simulink model "Noa_Nofusion"  (R2020b)
settings: Solver=FixedStepDiscrete  StartTime=0.0  StopTime=Inf  FixedStep=0.01  RelTol=1e-3
PostLoadFcn:
  | if any(exist('dsrtsu_mdlpostloadfcn', 'file') ~= 0), dsrtsu_mdlpostloadfcn('Execute', bdroot); end
InitFcn:
  | , if any(exist('rtifpga_mdlclblib', 'file') ~= 0), rtifpga_mdlclblib('Init', bdroot); end,
  | , if any(exist('dsmpb_private', 'file') ~= 0), dsmpb_private('dsmpb_mdlclblib', 'Init', bdroot); end,
undefined symbols (not defined in the file or in its folder): ACC_TimeGap_DecSetSwt, ACC_TimeGap_IncSetSwt, AccelPedalPosn, AccelPedalPosnVldty, AccelPedlPosnDiagc, AccPedalOverride, ACU_ShiftInProgress, ADAS_Posn_CurLane, AESSwtReq, ALC_SwtReq, BrkPedalSts, CC_ACC_CANCEL_OFFSwt, CC_ACC_CRUISE_OFFSwt, CC_ACC_DecSetSpd_SetSwt, CC_ACC_IncSetSpd_ResuSwt, CC_ACCSwtErr, CharSpd_ms, CSA_NODE, CURRENT_GEAR, CurrentGearValid, DiscIntNeverNeededParam, DrvDoorSts, DrvSBR, DrvTrqReqOvld, ECMACCInterface, ECMRespACC, ELKSwtReq, EngLimpHomeSts, EngSpd, EngState, EngState_PHEV, EngTrqMaxActSpd, EngTrqMinAct, EPS_DrvInpTrqVal_HighReslolution, EPS_FailSts, EPS_LKATorqOvrlDlvd, EPS_LKATorqOvrlDlvdVld, EPS_LKATrqOvlDlvdSts, EPS_SteerMod, EPS_TrqSnsrSts, EQ4_APPINFO, EQ4_LA_ELEM, EQ4_LA_HDR, EQ4_LAP_ELEM, EQ4_LAP_HDR, EQ4_LH_ELEM, EQ4_LH_HDR, EQ4_LRE_ELEM, EQ4_LRE_HDR, ESS_PedSwtReq, ESS_VehSwtReq, FFogLmpSts_F_Pbox, FLWheelDriveDirection, FLWheelSpd, FrntWiprSwtSts, FrntWshrSwtSts, FRWheelDriveDirection, FRWheelSpd, HazardLmpSwtSts, HCU_AccelPedalPosn_Diag ... (+151)
libraries: simulink x144, dsmpblib x33, canfdmsglib x10
(part 14 of 20)

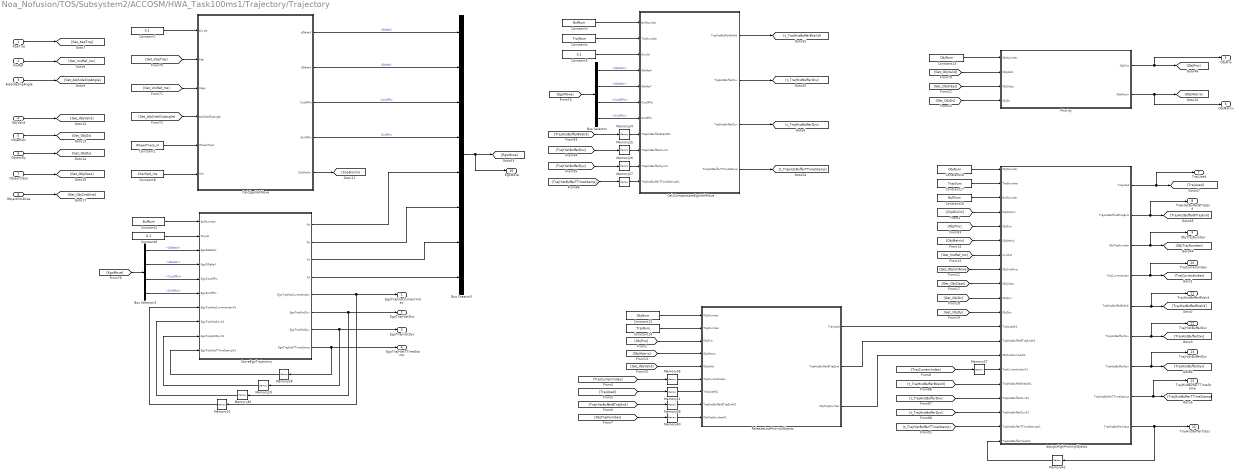
== system Noa_Nofusion/TOS/Subsystem2/ACCOSM/HWA_Task100ms1/Trajectory/Trajectory ==
  KapTraj : Inport
  VxvRef : Inport  Port=2
  AlpSideSlipAngle : Inport  Port=3
  ObjValid : Inport  Port=4
  ObjectDx : Inport  Port=5
  ObjectDy : Inport  Port=6
  ObjectClass : Inport  Port=7
  ObjectCntAlive : Inport  Port=8
  AssignHighPriorityObjects : MATLAB Function  TreatAsAtomicUnit=on
  Bus Creator3 : BusCreator  Inputs=8
  Bus Selector : BusSelector  OutputSignals=dDeltaX,dDeltaY,CosOfPsi,SinOfPsi
  Bus Selector3 : BusSelector  OutputSignals=dDeltaX,dDeltaY,CosOfPsi,SinOfPsi
  CalcCompensateEgoVehMove : MATLAB Function  TreatAsAtomicUnit=on
  CalcEgoVehMove : MATLAB Function  TreatAsAtomicUnit=on
  Constant1 : Constant  Value=WheelTrack_m  OutDataTypeStr=single
  Constant13 : Constant  Value=ObjNum  OutDataTypeStr=uint8
  Constant14 : Constant  Value=TrajNum  OutDataTypeStr=uint8
  Constant15 : Constant  Value=ObjNum  OutDataTypeStr=uint8
  Constant16 : Constant  Value=BufNum  OutDataTypeStr=uint8
  Constant17 : Constant  Value=TrajNum  OutDataTypeStr=uint8
  Constant18 : Constant  Value=ObjNum  OutDataTypeStr=uint8
  Constant2 : Constant  Value=BufNum  OutDataTypeStr=uint8
  Constant3 : Constant  Value=BufNum  OutDataTypeStr=uint8
  Constant4 : Constant  Value=TrajNum  OutDataTypeStr=uint8
  Constant5 : Constant  Value=0.1  OutDataTypeStr=single
  Constant6 : Constant  Value=0.1  OutDataTypeStr=single
  Constant7 : Constant  Value=0.1  OutDataTypeStr=single
  Constant8 : Constant  Value=CharSpd_ms  OutDataTypeStr=single
  Memory{24..26,42} (4 alike) : Memory  InitialCondition=zeros(TrajNum,BufNum)  InheritSampleTime=on
  Memory27 : Memory  InitialCondition=32*ones(TrajNum,BufNum)  InheritSampleTime=on
  Memory28 : Memory  InitialCondition=32*ones(BufNum,1)  InheritSampleTime=on
  Memory29 : Memory  InitialCondition=zeros(BufNum,1)  InheritSampleTime=on
  Memory30 : Memory  InitialCondition=zeros(BufNum,1)  InheritSampleTime=on
  Memory31 : Memory  InitialCondition=1  InheritSampleTime=on
  Memory36 : Memory  InitialCondition=ones(TrajNum,1)  InheritSampleTime=on
  Memory37 : Memory  InitialCondition=ones(TrajNum,1)  InheritSampleTime=on
  Memory38 : Memory  InitialCondition=ones(TrajNum,BufNum)  InheritSampleTime=on
  Memory40 : Memory  InitialCondition=255*ones(ObjNum,1)  InheritSampleTime=on
  Memory41 : Memory  InitialCondition=zeros(TrajNum,1)  InheritSampleTime=on
  Priority : MATLAB Function  TreatAsAtomicUnit=on
  ReleaseLowPriorityObjects : MATLAB Function  TreatAsAtomicUnit=on
  StoreEgoTrajectory : MATLAB Function  TreatAsAtomicUnit=on
  EgoTrajHistCurrentIndex : Outport
  EgoTrajHistDxv : Outport  Port=2
  EgoTrajHistDyv : Outport  Port=3
  EgoTrajHistTTimeStamp : Outport  Port=4
  ObjPrio : Outport  Port=5
  ObjMatrix : Outport  Port=6
  TrajUsed : Outport  Port=7
  TrajHistBufferBTrajEnd : Outport  Port=8
  ObjTrajNumber : Outport  Port=9
  TrajCurrentIndex : Outport  Port=10
  TrajHistBufferBValid : Outport  Port=11
  TrajHistBufferDxv : Outport  Port=12
  TrajHistBufferDyv : Outport  Port=13
  TrajHistBufferTTimeStamp : Outport  Port=14
  TrajHistBufferClass : Outport  Port=15
  EgoMove : Outport  Port=16
  wires:
  StoreEgoTrajectory/1(Pa) -> Bus Creator3/5
  StoreEgoTrajectory/2(Pb) -> Bus Creator3/6
  StoreEgoTrajectory/3(Pc) -> Bus Creator3/7
  StoreEgoTrajectory/4(Pd) -> Bus Creator3/8
  Bus Creator3/1 -> [EgoMove], EgoMove/1
  [SlipDislim] -> AssignHighPriorityObjects/4(SlipDisLim)
  CalcEgoVehMove/5(SlipDislim) -> [SlipDislim]
  Constant8/1 -> CalcEgoVehMove/6(Vch)
  Constant1/1 -> CalcEgoVehMove/5(WheelTrack)
  CalcCompensateEgoVehMove/3(TrajHistBufferDyv) -> [t_TrajHistBufferDyv]
  Priority/2(ObjMatrix) -> ObjMatrix/1, [ObjMatrix]
  Priority/1(ObjPrio) -> [ObjPrio], ObjPrio/1
  CalcEgoVehMove/4(SinOfPsi) -> Bus Creator3/4  "SinOfPsi"
  CalcEgoVehMove/3(CosOfPsi) -> Bus Creator3/3  "CosOfPsi"
  CalcEgoVehMove/2(dDeltaY) -> Bus Creator3/2  "dDeltaY"
  CalcEgoVehMove/1(dDeltaX) -> Bus Creator3/1  "dDeltaX"
  ObjectCntAlive/1 -> [Get_ObjCntAlive]
  ObjectClass/1 -> [Get_ObjClass]
  ObjectDx/1 -> [Get_ObjDx]
  ObjectDy/1 -> [Get_ObjDy]
  ObjValid/1 -> [Get_ObjValid]
  AssignHighPriorityObjects/8(TrajHistBufferTTimeStamp) -> [TrajHistBufferTTimeStamp], TrajHistBufferTTimeStamp/1
  Bus Selector3/1 -> StoreEgoTrajectory/3(EgoDDeltaX)  "<dDeltaX>"
  Bus Selector3/4 -> StoreEgoTrajectory/6(EgoSinOfPsi)  "<SinOfPsi>"
  Bus Selector3/2 -> StoreEgoTrajectory/4(EgoDDeltaY)  "<dDeltaY>"
  Bus Selector3/3 -> StoreEgoTrajectory/5(EgoCosOfPsi)  "<CosOfPsi>"
  StoreEgoTrajectory/8(EgoTrajHistTTimeStamp) -> Memory28/1, EgoTrajHistTTimeStamp/1
  Memory31/1 -> StoreEgoTrajectory/7(EgoTrajHistCurrentIndexK1)
  StoreEgoTrajectory/5(EgoTrajHistCurrentIndex) -> Memory31/1, EgoTrajHistCurrentIndex/1
  Memory30/1 -> StoreEgoTrajectory/8(EgoTrajHistDxvK1)
  StoreEgoTrajectory/6(EgoTrajHistDxv) -> Memory30/1, EgoTrajHistDxv/1
  Memory29/1 -> StoreEgoTrajectory/9(EgoTrajHistDyvK1)
  Memory28/1 -> StoreEgoTrajectory/10(EgoTrajHistTTimeStampK1)
  StoreEgoTrajectory/7(EgoTrajHistDyv) -> Memory29/1, EgoTrajHistDyv/1
  Constant6/1 -> StoreEgoTrajectory/2(tCycle)
  Constant2/1 -> StoreEgoTrajectory/1(BufNumber)
  [ObjMatrix] -> AssignHighPriorityObjects/6(ObjMatrix)
  [ObjMatrix] -> ReleaseLowPriorityObjects/4(ObjMatrix)
  Constant16/1 -> AssignHighPriorityObjects/3(BufNumber)
  Constant17/1 -> AssignHighPriorityObjects/2(TrajNumber)
  Constant18/1 -> AssignHighPriorityObjects/1(ObjNumber)
  Constant14/1 -> ReleaseLowPriorityObjects/2(TrajNumber)
  Constant15/1 -> ReleaseLowPriorityObjects/1(ObjNumber)
  Constant13/1 -> Priority/1(ObjNumber)
  Constant4/1 -> CalcCompensateEgoVehMove/2(TrajNumber)
  Constant3/1 -> CalcCompensateEgoVehMove/1(BufNumber)
  AlpSideSlipAngle/1 -> [Get_AlpSideSlipAngle]
  VxvRef/1 -> [Get_VxvRef_ms]
  KapTraj/1 -> [Get_KapTraj]
  [Get_ObjCntAlive] -> AssignHighPriorityObjects/8(ObjCntAlive)
  [TrajHistBufferBValid] -> Memory24/1
  [TrajHistBufferDyv] -> Memory26/1
  [TrajHistBufferDxv] -> Memory25/1
  [TrajHistBufferTTimeStamp] -> Memory27/1
  [Get_ObjDy] -> AssignHighPriorityObjects/11(ObjDyv)
  AssignHighPriorityObjects/4(TrajCurrentIndex) -> [TrajCurrentIndex], TrajCurrentIndex/1
  [Get_ObjDx] -> AssignHighPriorityObjects/10(ObjDxv)
  [Get_ObjClass] -> AssignHighPriorityObjects/9(ObjClass)
  [Get_VxvRef_ms] -> AssignHighPriorityObjects/7(VxvRef)
  [TrajCurrentIndex] -> Memory37/1
  [TrajCurrentIndex] -> Memory36/1
  AssignHighPriorityObjects/6(TrajHistBufferDxv) -> [TrajHistBufferDxv], TrajHistBufferDxv/1
  AssignHighPriorityObjects/7(TrajHistBufferDyv) -> [TrajHistBufferDyv], TrajHistBufferDyv/1
  AssignHighPriorityObjects/5(TrajHistBufferBValid) -> [TrajHistBufferBValid], TrajHistBufferBValid/1
  [Get_ObjValid] -> ReleaseLowPriorityObjects/5(ObjValid)
  [ObjPrio] -> ReleaseLowPriorityObjects/3(ObjPrio)
  [TrajHistBufferBTrajEnd] -> Memory38/1
  [ObjTrajNumber] -> Memory40/1
  [TrajUsed] -> Memory41/1
  Memory42/1 -> AssignHighPriorityObjects/20(TrajHistBufferClassK1)
  Memory41/1 -> ReleaseLowPriorityObjects/7(TrajUsedK1)
  Memory40/1 -> ReleaseLowPriorityObjects/9(ObjTrajNumberK1)
  Memory38/1 -> ReleaseLowPriorityObjects/8(TrajHistBufferBTrajEndK1)
  Memory37/1 -> AssignHighPriorityObjects/15(TrajCurrentIndexK1)
  Memory36/1 -> ReleaseLowPriorityObjects/6(TrajCurrentIndex)
  [t_TrajHistBufferTTimeStamp] -> AssignHighPriorityObjects/19(TrajHistBufferTTimeStampK1)
  CalcCompensateEgoVehMove/4(TrajHistBufferTTimeStamp) -> [t_TrajHistBufferTTimeStamp]
  [t_TrajHistBufferDyv] -> AssignHighPriorityObjects/18(TrajHistBufferDyvK1)
  [t_TrajHistBufferDxv] -> AssignHighPriorityObjects/17(TrajHistBufferDxvK1)
  CalcCompensateEgoVehMove/2(TrajHistBufferDxv) -> [t_TrajHistBufferDxv]
  [t_TrajHistBufferBValid] -> AssignHighPriorityObjects/16(TrajHistBufferBValidK1)
  CalcCompensateEgoVehMove/1(TrajHistBufferBValid) -> [t_TrajHistBufferBValid]
  [ObjPrio] -> AssignHighPriorityObjects/5(ObjPrio)
  AssignHighPriorityObjects/9(TrajHistBufferClass) -> TrajHistBufferClass/1, Memory42/1
  AssignHighPriorityObjects/2(TrajHistBufferBTrajEnd) -> [TrajHistBufferBTrajEnd], TrajHistBufferBTrajEnd/1
  AssignHighPriorityObjects/1(TrajUsed) -> [TrajUsed], TrajUsed/1
  ReleaseLowPriorityObjects/3(ObjTrajNumber) -> AssignHighPriorityObjects/14(ObjTrajNumberK1)
  AssignHighPriorityObjects/3(ObjTrajNumber) -> [ObjTrajNumber], ObjTrajNumber/1
  ReleaseLowPriorityObjects/1(TrajUsed) -> AssignHighPriorityObjects/12(TrajUsedK1)
  ReleaseLowPriorityObjects/2(TrajHistBufferBTrajEnd) -> AssignHighPriorityObjects/13(TrajHistBufferBTrajEndK1)
  [Get_ObjValid] -> Priority/2(ObjValid)
  [Get_ObjClass] -> Priority/3(ObjClass)
  [Get_ObjDx] -> Priority/4(ObjDx)
  [EgoMove] -> Bus Selector3/1
  Bus Selector/4 -> CalcCompensateEgoVehMove/7(SinOfPsi)  "<SinOfPsi>"
  Bus Selector/3 -> CalcCompensateEgoVehMove/6(CosOfPsi)  "<CosOfPsi>"
  Bus Selector/2 -> CalcCompensateEgoVehMove/5(dDeltaY)  "<dDeltaY>"
  Bus Selector/1 -> CalcCompensateEgoVehMove/4(dDeltaX)  "<dDeltaX>"
  [EgoMove] -> Bus Selector/1
  Memory27/1 -> CalcCompensateEgoVehMove/11(TrajHistBufferTTimeStampK1)
  Memory26/1 -> CalcCompensateEgoVehMove/10(TrajHistBufferDyvK1)
  Memory25/1 -> CalcCompensateEgoVehMove/9(TrajHistBufferDxvK1)
  Memory24/1 -> CalcCompensateEgoVehMove/8(TrajHistBufferBValidK1)
  Constant5/1 -> CalcCompensateEgoVehMove/3(tCycle)
  [Get_KapTraj] -> CalcEgoVehMove/2(Kap)
  [Get_AlpSideSlipAngle] -> CalcEgoVehMove/4(alpSideSlipAngle)
  [Get_VxvRef_ms] -> CalcEgoVehMove/3(Vego)
  Constant7/1 -> CalcEgoVehMove/1(tCycle)

== system Noa_Nofusion/TOS/Subsystem2/ACCOSM/ObjMatrixTransit/Subsystem/For Each Subsystem ==
  <EQ4_OBJ_ELEM> : Inport  Partition=on  PartitionDimension=1  PartitionWidth=1  PartitionOffset=0
  Bus Selector : BusSelector  OutputSignals=OBJ_ID,OBJ_Existence_Probability,OBJ_Object_Class,OBJ_Width,OBJ_Long_Distance,OBJ_Lat_Distance,OBJ_Abs_Long_Acc,OBJ_Abs_Long_Velocity,OBJ_Abs_Lat_Velocity,OBJ_Brake_Light,OBJ_Object_Age,OBJ_Motion_Status,OBJ_Motion_Category,OBJ_Motion_Orientation
  For Each : ForEach  DisableCoverage=on
  id : Outport  ConcatenationDimension=1
  confidence : Outport  Port=2  ConcatenationDimension=1
  classification : Outport  Port=3  ConcatenationDimension=1
  width : Outport  Port=4  ConcatenationDimension=1
  LongDis : Outport  Port=5  ConcatenationDimension=1
  LatDis : Outport  Port=6  ConcatenationDimension=1
  AbsLongAcc : Outport  Port=7  ConcatenationDimension=1
  AbsLongVel : Outport  Port=8  ConcatenationDimension=1
  AbsLatVel : Outport  Port=9  ConcatenationDimension=1
  BrakeLight : Outport  Port=10  ConcatenationDimension=1
  Age : Outport  Port=11  ConcatenationDimension=1
  motionSts : Outport  Port=12  ConcatenationDimension=1
  motionCategory : Outport  Port=13  ConcatenationDimension=1
  motionOrientation : Outport  Port=14  ConcatenationDimension=1
  wires:
  <EQ4_OBJ_ELEM>/1 -> Bus Selector/1
  Bus Selector/12 -> motionSts/1  "<OBJ_Motion_Status>"
  Bus Selector/6 -> LatDis/1  "<OBJ_Lat_Distance>"
  Bus Selector/9 -> AbsLatVel/1  "<OBJ_Abs_Lat_Velocity>"
  Bus Selector/7 -> AbsLongAcc/1  "<OBJ_Abs_Long_Acc>"
  Bus Selector/1 -> id/1  "<OBJ_ID>"
  Bus Selector/2 -> confidence/1  "<OBJ_Existence_Probability>"
  Bus Selector/10 -> BrakeLight/1  "<OBJ_Brake_Light>"
  Bus Selector/8 -> AbsLongVel/1  "<OBJ_Abs_Long_Velocity>"
  Bus Selector/5 -> LongDis/1  "<OBJ_Long_Distance>"
  Bus Selector/11 -> Age/1  "<OBJ_Object_Age>"
  Bus Selector/4 -> width/1  "<OBJ_Width>"
  Bus Selector/14 -> motionOrientation/1  "<OBJ_Motion_Orientation>"
  Bus Selector/3 -> classification/1  "<OBJ_Object_Class>"
  Bus Selector/13 -> motionCategory/1  "<OBJ_Motion_Category>"

== system Noa_Nofusion/TOS/Subsystem2/ACCOSM/ObjMatrixTransit/Subsystem/For Iterator Subsystem ==
  <EQ4_OBJ_ELEM> : Inport
  Bus Selector : BusSelector  OutputSignals=OBJ_ID,OBJ_Existence_Probability,OBJ_Object_Class,OBJ_Width,OBJ_Long_Distance,OBJ_Lat_Distance,OBJ_Abs_Long_Acc,OBJ_Abs_Long_Velocity,OBJ_Abs_Lat_Velocity,OBJ_Brake_Light,OBJ_Object_Age,OBJ_Motion_Status,OBJ_Motion_Category,OBJ_Motion_Orientation
  For Iterator : ForIterator  IterationLimit=20
  Selector : Selector  InputPortWidth=20  IndexOptions=Index vector (port)  Indices=[1 3]  OutputSizes=1
  id : Outport
  confidence : Outport  Port=2
  classification : Outport  Port=3
  width : Outport  Port=4
  LongDis : Outport  Port=5
  LatDis : Outport  Port=6
  AbsLongAcc : Outport  Port=7
  AbsLongVel : Outport  Port=8
  AbsLatVel : Outport  Port=9
  BrakeLight : Outport  Port=10
  Age : Outport  Port=11
  motionSts : Outport  Port=12
  motionCategory : Outport  Port=13
  motionOrientation : Outport  Port=14
  wires:
  <EQ4_OBJ_ELEM>/1 -> Selector/1
  For Iterator/1 -> Selector/2
  Selector/1 -> Bus Selector/1
  Bus Selector/1 -> id/1  "<OBJ_ID>"
  Bus Selector/2 -> confidence/1  "<OBJ_Existence_Probability>"
  Bus Selector/3 -> classification/1  "<OBJ_Object_Class>"
  Bus Selector/4 -> width/1  "<OBJ_Width>"
  Bus Selector/5 -> LongDis/1  "<OBJ_Long_Distance>"
  Bus Selector/6 -> LatDis/1  "<OBJ_Lat_Distance>"
  Bus Selector/7 -> AbsLongAcc/1  "<OBJ_Abs_Long_Acc>"
  Bus Selector/8 -> AbsLongVel/1  "<OBJ_Abs_Long_Velocity>"
  Bus Selector/9 -> AbsLatVel/1  "<OBJ_Abs_Lat_Velocity>"
  Bus Selector/10 -> BrakeLight/1  "<OBJ_Brake_Light>"
  Bus Selector/11 -> Age/1  "<OBJ_Object_Age>"
  Bus Selector/12 -> motionSts/1  "<OBJ_Motion_Status>"
  Bus Selector/13 -> motionCategory/1  "<OBJ_Motion_Category>"
  Bus Selector/14 -> motionOrientation/1  "<OBJ_Motion_Orientation>"

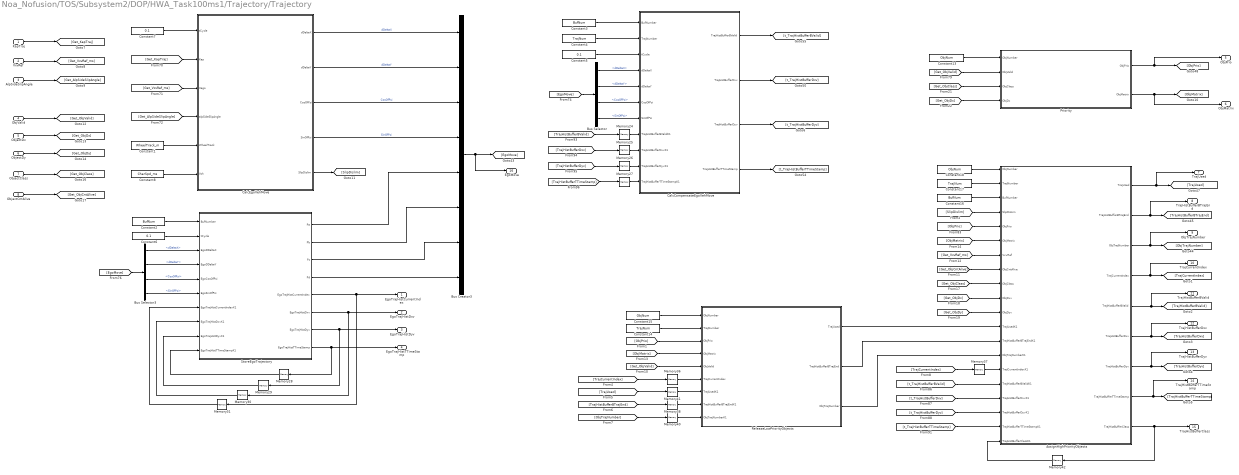
== system Noa_Nofusion/TOS/Subsystem2/DOP/HWA_Task100ms1/Trajectory/Trajectory ==
  KapTraj : Inport
  VxvRef : Inport  Port=2
  AlpSideSlipAngle : Inport  Port=3
  ObjValid : Inport  Port=4
  ObjectDx : Inport  Port=5
  ObjectDy : Inport  Port=6
  ObjectClass : Inport  Port=7
  ObjectCntAlive : Inport  Port=8
  AssignHighPriorityObjects : MATLAB Function  TreatAsAtomicUnit=on
  Bus Creator3 : BusCreator  Inputs=8
  Bus Selector : BusSelector  OutputSignals=dDeltaX,dDeltaY,CosOfPsi,SinOfPsi
  Bus Selector3 : BusSelector  OutputSignals=dDeltaX,dDeltaY,CosOfPsi,SinOfPsi
  CalcCompensateEgoVehMove : MATLAB Function  TreatAsAtomicUnit=on
  CalcEgoVehMove : MATLAB Function  TreatAsAtomicUnit=on
  Constant1 : Constant  Value=WheelTrack_m  OutDataTypeStr=single
  Constant13 : Constant  Value=ObjNum  OutDataTypeStr=uint8
  Constant14 : Constant  Value=TrajNum  OutDataTypeStr=uint8
  Constant15 : Constant  Value=ObjNum  OutDataTypeStr=uint8
  Constant16 : Constant  Value=BufNum  OutDataTypeStr=uint8
  Constant17 : Constant  Value=TrajNum  OutDataTypeStr=uint8
  Constant18 : Constant  Value=ObjNum  OutDataTypeStr=uint8
  Constant2 : Constant  Value=BufNum  OutDataTypeStr=uint8
  Constant3 : Constant  Value=BufNum  OutDataTypeStr=uint8
  Constant4 : Constant  Value=TrajNum  OutDataTypeStr=uint8
  Constant5 : Constant  Value=0.1  OutDataTypeStr=single
  Constant6 : Constant  Value=0.1  OutDataTypeStr=single
  Constant7 : Constant  Value=0.1  OutDataTypeStr=single
  Constant8 : Constant  Value=CharSpd_ms  OutDataTypeStr=single
  Memory{24..26,42} (4 alike) : Memory  InitialCondition=zeros(TrajNum,BufNum)  InheritSampleTime=on
  Memory27 : Memory  InitialCondition=32*ones(TrajNum,BufNum)  InheritSampleTime=on
  Memory28 : Memory  InitialCondition=32*ones(BufNum,1)  InheritSampleTime=on
  Memory29 : Memory  InitialCondition=zeros(BufNum,1)  InheritSampleTime=on
  Memory30 : Memory  InitialCondition=zeros(BufNum,1)  InheritSampleTime=on
  Memory31 : Memory  InitialCondition=1  InheritSampleTime=on
  Memory36 : Memory  InitialCondition=ones(TrajNum,1)  InheritSampleTime=on
  Memory37 : Memory  InitialCondition=ones(TrajNum,1)  InheritSampleTime=on
  Memory38 : Memory  InitialCondition=ones(TrajNum,BufNum)  InheritSampleTime=on
  Memory40 : Memory  InitialCondition=255*ones(ObjNum,1)  InheritSampleTime=on
  Memory41 : Memory  InitialCondition=zeros(TrajNum,1)  InheritSampleTime=on
  Priority : MATLAB Function  TreatAsAtomicUnit=on
  ReleaseLowPriorityObjects : MATLAB Function  TreatAsAtomicUnit=on
  StoreEgoTrajectory : MATLAB Function  TreatAsAtomicUnit=on
  EgoTrajHistCurrentIndex : Outport
  EgoTrajHistDxv : Outport  Port=2
  EgoTrajHistDyv : Outport  Port=3
  EgoTrajHistTTimeStamp : Outport  Port=4
  ObjPrio : Outport  Port=5
  ObjMatrix : Outport  Port=6
  TrajUsed : Outport  Port=7
  TrajHistBufferBTrajEnd : Outport  Port=8
  ObjTrajNumber : Outport  Port=9
  TrajCurrentIndex : Outport  Port=10
  TrajHistBufferBValid : Outport  Port=11
  TrajHistBufferDxv : Outport  Port=12
  TrajHistBufferDyv : Outport  Port=13
  TrajHistBufferTTimeStamp : Outport  Port=14
  TrajHistBufferClass : Outport  Port=15
  EgoMove : Outport  Port=16
  wires:
  Constant7/1 -> CalcEgoVehMove/1(tCycle)
  [Get_VxvRef_ms] -> CalcEgoVehMove/3(Vego)
  [Get_AlpSideSlipAngle] -> CalcEgoVehMove/4(alpSideSlipAngle)
  [Get_KapTraj] -> CalcEgoVehMove/2(Kap)
  Constant5/1 -> CalcCompensateEgoVehMove/3(tCycle)
  Memory24/1 -> CalcCompensateEgoVehMove/8(TrajHistBufferBValidK1)
  Memory25/1 -> CalcCompensateEgoVehMove/9(TrajHistBufferDxvK1)
  Memory26/1 -> CalcCompensateEgoVehMove/10(TrajHistBufferDyvK1)
  Memory27/1 -> CalcCompensateEgoVehMove/11(TrajHistBufferTTimeStampK1)
  [EgoMove] -> Bus Selector/1
  Bus Selector/1 -> CalcCompensateEgoVehMove/4(dDeltaX)  "<dDeltaX>"
  Bus Selector/2 -> CalcCompensateEgoVehMove/5(dDeltaY)  "<dDeltaY>"
  Bus Selector/3 -> CalcCompensateEgoVehMove/6(CosOfPsi)  "<CosOfPsi>"
  Bus Selector/4 -> CalcCompensateEgoVehMove/7(SinOfPsi)  "<SinOfPsi>"
  [EgoMove] -> Bus Selector3/1
  [Get_ObjDx] -> Priority/4(ObjDx)
  [Get_ObjClass] -> Priority/3(ObjClass)
  [Get_ObjValid] -> Priority/2(ObjValid)
  ReleaseLowPriorityObjects/2(TrajHistBufferBTrajEnd) -> AssignHighPriorityObjects/13(TrajHistBufferBTrajEndK1)
  ReleaseLowPriorityObjects/1(TrajUsed) -> AssignHighPriorityObjects/12(TrajUsedK1)
  AssignHighPriorityObjects/3(ObjTrajNumber) -> ObjTrajNumber/1, [ObjTrajNumber]
  ReleaseLowPriorityObjects/3(ObjTrajNumber) -> AssignHighPriorityObjects/14(ObjTrajNumberK1)
  AssignHighPriorityObjects/1(TrajUsed) -> TrajUsed/1, [TrajUsed]
  AssignHighPriorityObjects/2(TrajHistBufferBTrajEnd) -> TrajHistBufferBTrajEnd/1, [TrajHistBufferBTrajEnd]
  AssignHighPriorityObjects/9(TrajHistBufferClass) -> Memory42/1, TrajHistBufferClass/1
  [ObjPrio] -> AssignHighPriorityObjects/5(ObjPrio)
  CalcCompensateEgoVehMove/1(TrajHistBufferBValid) -> [t_TrajHistBufferBValid]
  [t_TrajHistBufferBValid] -> AssignHighPriorityObjects/16(TrajHistBufferBValidK1)
  CalcCompensateEgoVehMove/2(TrajHistBufferDxv) -> [t_TrajHistBufferDxv]
  [t_TrajHistBufferDxv] -> AssignHighPriorityObjects/17(TrajHistBufferDxvK1)
  [t_TrajHistBufferDyv] -> AssignHighPriorityObjects/18(TrajHistBufferDyvK1)
  CalcCompensateEgoVehMove/4(TrajHistBufferTTimeStamp) -> [t_TrajHistBufferTTimeStamp]
  [t_TrajHistBufferTTimeStamp] -> AssignHighPriorityObjects/19(TrajHistBufferTTimeStampK1)
  Memory36/1 -> ReleaseLowPriorityObjects/6(TrajCurrentIndex)
  Memory37/1 -> AssignHighPriorityObjects/15(TrajCurrentIndexK1)
  Memory38/1 -> ReleaseLowPriorityObjects/8(TrajHistBufferBTrajEndK1)
  Memory40/1 -> ReleaseLowPriorityObjects/9(ObjTrajNumberK1)
  Memory41/1 -> ReleaseLowPriorityObjects/7(TrajUsedK1)
  Memory42/1 -> AssignHighPriorityObjects/20(TrajHistBufferClassK1)
  [TrajUsed] -> Memory41/1
  [ObjTrajNumber] -> Memory40/1
  [TrajHistBufferBTrajEnd] -> Memory38/1
  [ObjPrio] -> ReleaseLowPriorityObjects/3(ObjPrio)
  [Get_ObjValid] -> ReleaseLowPriorityObjects/5(ObjValid)
  AssignHighPriorityObjects/5(TrajHistBufferBValid) -> TrajHistBufferBValid/1, [TrajHistBufferBValid]
  AssignHighPriorityObjects/7(TrajHistBufferDyv) -> TrajHistBufferDyv/1, [TrajHistBufferDyv]
  AssignHighPriorityObjects/6(TrajHistBufferDxv) -> TrajHistBufferDxv/1, [TrajHistBufferDxv]
  [TrajCurrentIndex] -> Memory36/1
  [TrajCurrentIndex] -> Memory37/1
  [Get_VxvRef_ms] -> AssignHighPriorityObjects/7(VxvRef)
  [Get_ObjClass] -> AssignHighPriorityObjects/9(ObjClass)
  [Get_ObjDx] -> AssignHighPriorityObjects/10(ObjDxv)
  AssignHighPriorityObjects/4(TrajCurrentIndex) -> TrajCurrentIndex/1, [TrajCurrentIndex]
  [Get_ObjDy] -> AssignHighPriorityObjects/11(ObjDyv)
  [TrajHistBufferTTimeStamp] -> Memory27/1
  [TrajHistBufferDxv] -> Memory25/1
  [TrajHistBufferDyv] -> Memory26/1
  [TrajHistBufferBValid] -> Memory24/1
  [Get_ObjCntAlive] -> AssignHighPriorityObjects/8(ObjCntAlive)
  KapTraj/1 -> [Get_KapTraj]
  VxvRef/1 -> [Get_VxvRef_ms]
  AlpSideSlipAngle/1 -> [Get_AlpSideSlipAngle]
  Constant3/1 -> CalcCompensateEgoVehMove/1(BufNumber)
  Constant4/1 -> CalcCompensateEgoVehMove/2(TrajNumber)
  Constant13/1 -> Priority/1(ObjNumber)
  Constant15/1 -> ReleaseLowPriorityObjects/1(ObjNumber)
  Constant14/1 -> ReleaseLowPriorityObjects/2(TrajNumber)
  Constant18/1 -> AssignHighPriorityObjects/1(ObjNumber)
  Constant17/1 -> AssignHighPriorityObjects/2(TrajNumber)
  Constant16/1 -> AssignHighPriorityObjects/3(BufNumber)
  [ObjMatrix] -> ReleaseLowPriorityObjects/4(ObjMatrix)
  [ObjMatrix] -> AssignHighPriorityObjects/6(ObjMatrix)
  Constant2/1 -> StoreEgoTrajectory/1(BufNumber)
  Constant6/1 -> StoreEgoTrajectory/2(tCycle)
  StoreEgoTrajectory/7(EgoTrajHistDyv) -> EgoTrajHistDyv/1, Memory29/1
  Memory28/1 -> StoreEgoTrajectory/10(EgoTrajHistTTimeStampK1)
  Memory29/1 -> StoreEgoTrajectory/9(EgoTrajHistDyvK1)
  StoreEgoTrajectory/6(EgoTrajHistDxv) -> EgoTrajHistDxv/1, Memory30/1
  Memory30/1 -> StoreEgoTrajectory/8(EgoTrajHistDxvK1)
  StoreEgoTrajectory/5(EgoTrajHistCurrentIndex) -> EgoTrajHistCurrentIndex/1, Memory31/1
  Memory31/1 -> StoreEgoTrajectory/7(EgoTrajHistCurrentIndexK1)
  StoreEgoTrajectory/8(EgoTrajHistTTimeStamp) -> EgoTrajHistTTimeStamp/1, Memory28/1
  Bus Selector3/3 -> StoreEgoTrajectory/5(EgoCosOfPsi)  "<CosOfPsi>"
  Bus Selector3/2 -> StoreEgoTrajectory/4(EgoDDeltaY)  "<dDeltaY>"
  Bus Selector3/4 -> StoreEgoTrajectory/6(EgoSinOfPsi)  "<SinOfPsi>"
  Bus Selector3/1 -> StoreEgoTrajectory/3(EgoDDeltaX)  "<dDeltaX>"
  AssignHighPriorityObjects/8(TrajHistBufferTTimeStamp) -> TrajHistBufferTTimeStamp/1, [TrajHistBufferTTimeStamp]
  ObjValid/1 -> [Get_ObjValid]
  ObjectDy/1 -> [Get_ObjDy]
  ObjectDx/1 -> [Get_ObjDx]
  ObjectClass/1 -> [Get_ObjClass]
  ObjectCntAlive/1 -> [Get_ObjCntAlive]
  CalcEgoVehMove/1(dDeltaX) -> Bus Creator3/1  "dDeltaX"
  CalcEgoVehMove/2(dDeltaY) -> Bus Creator3/2  "dDeltaY"
  CalcEgoVehMove/3(CosOfPsi) -> Bus Creator3/3  "CosOfPsi"
  CalcEgoVehMove/4(SinOfPsi) -> Bus Creator3/4  "SinOfPsi"
  Priority/1(ObjPrio) -> ObjPrio/1, [ObjPrio]
  Priority/2(ObjMatrix) -> [ObjMatrix], ObjMatrix/1
  CalcCompensateEgoVehMove/3(TrajHistBufferDyv) -> [t_TrajHistBufferDyv]
  Constant1/1 -> CalcEgoVehMove/5(WheelTrack)
  Constant8/1 -> CalcEgoVehMove/6(Vch)
  CalcEgoVehMove/5(SlipDislim) -> [SlipDislim]
  [SlipDislim] -> AssignHighPriorityObjects/4(SlipDisLim)
  Bus Creator3/1 -> EgoMove/1, [EgoMove]
  StoreEgoTrajectory/4(Pd) -> Bus Creator3/8
  StoreEgoTrajectory/3(Pc) -> Bus Creator3/7
  StoreEgoTrajectory/2(Pb) -> Bus Creator3/6
  StoreEgoTrajectory/1(Pa) -> Bus Creator3/5

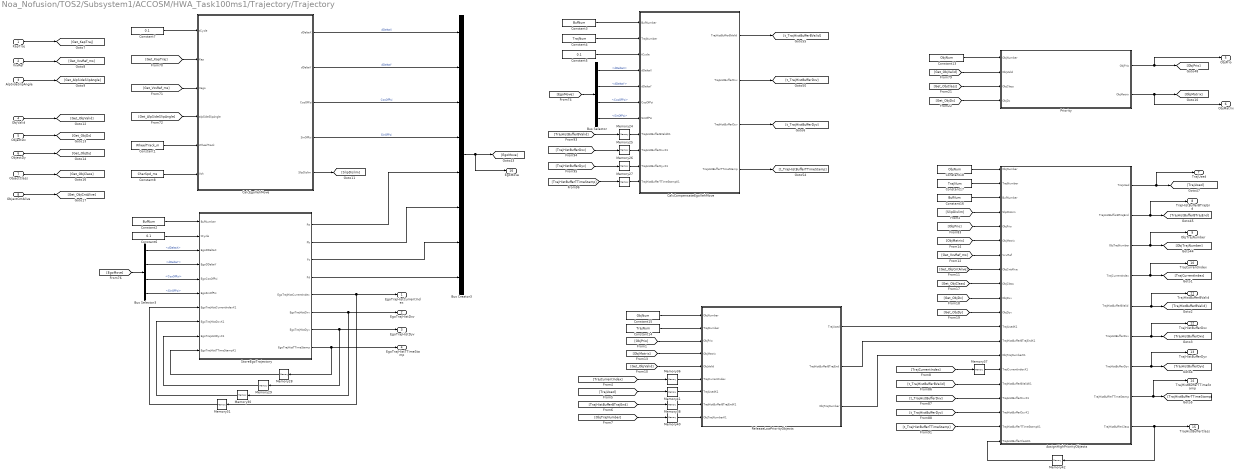
== system Noa_Nofusion/TOS2/Subsystem1/ACCOSM/HWA_Task100ms1/Trajectory/Trajectory ==
  KapTraj : Inport
  VxvRef : Inport  Port=2
  AlpSideSlipAngle : Inport  Port=3
  ObjValid : Inport  Port=4
  ObjectDx : Inport  Port=5
  ObjectDy : Inport  Port=6
  ObjectClass : Inport  Port=7
  ObjectCntAlive : Inport  Port=8
  AssignHighPriorityObjects : MATLAB Function  TreatAsAtomicUnit=on
  Bus Creator3 : BusCreator  Inputs=8
  Bus Selector : BusSelector  OutputSignals=dDeltaX,dDeltaY,CosOfPsi,SinOfPsi
  Bus Selector3 : BusSelector  OutputSignals=dDeltaX,dDeltaY,CosOfPsi,SinOfPsi
  CalcCompensateEgoVehMove : MATLAB Function  TreatAsAtomicUnit=on
  CalcEgoVehMove : MATLAB Function  TreatAsAtomicUnit=on
  Constant1 : Constant  Value=WheelTrack_m  OutDataTypeStr=single
  Constant13 : Constant  Value=ObjNum  OutDataTypeStr=uint8
  Constant14 : Constant  Value=TrajNum  OutDataTypeStr=uint8
  Constant15 : Constant  Value=ObjNum  OutDataTypeStr=uint8
  Constant16 : Constant  Value=BufNum  OutDataTypeStr=uint8
  Constant17 : Constant  Value=TrajNum  OutDataTypeStr=uint8
  Constant18 : Constant  Value=ObjNum  OutDataTypeStr=uint8
  Constant2 : Constant  Value=BufNum  OutDataTypeStr=uint8
  Constant3 : Constant  Value=BufNum  OutDataTypeStr=uint8
  Constant4 : Constant  Value=TrajNum  OutDataTypeStr=uint8
  Constant5 : Constant  Value=0.1  OutDataTypeStr=single
  Constant6 : Constant  Value=0.1  OutDataTypeStr=single
  Constant7 : Constant  Value=0.1  OutDataTypeStr=single
  Constant8 : Constant  Value=CharSpd_ms  OutDataTypeStr=single
  Memory{24..26,42} (4 alike) : Memory  InitialCondition=zeros(TrajNum,BufNum)  InheritSampleTime=on
  Memory27 : Memory  InitialCondition=32*ones(TrajNum,BufNum)  InheritSampleTime=on
  Memory28 : Memory  InitialCondition=32*ones(BufNum,1)  InheritSampleTime=on
  Memory29 : Memory  InitialCondition=zeros(BufNum,1)  InheritSampleTime=on
  Memory30 : Memory  InitialCondition=zeros(BufNum,1)  InheritSampleTime=on
  Memory31 : Memory  InitialCondition=1  InheritSampleTime=on
  Memory36 : Memory  InitialCondition=ones(TrajNum,1)  InheritSampleTime=on
  Memory37 : Memory  InitialCondition=ones(TrajNum,1)  InheritSampleTime=on
  Memory38 : Memory  InitialCondition=ones(TrajNum,BufNum)  InheritSampleTime=on
  Memory40 : Memory  InitialCondition=255*ones(ObjNum,1)  InheritSampleTime=on
  Memory41 : Memory  InitialCondition=zeros(TrajNum,1)  InheritSampleTime=on
  Priority : MATLAB Function  TreatAsAtomicUnit=on
  ReleaseLowPriorityObjects : MATLAB Function  TreatAsAtomicUnit=on
  StoreEgoTrajectory : MATLAB Function  TreatAsAtomicUnit=on
  EgoTrajHistCurrentIndex : Outport
  EgoTrajHistDxv : Outport  Port=2
  EgoTrajHistDyv : Outport  Port=3
  EgoTrajHistTTimeStamp : Outport  Port=4
  ObjPrio : Outport  Port=5
  ObjMatrix : Outport  Port=6
  TrajUsed : Outport  Port=7
  TrajHistBufferBTrajEnd : Outport  Port=8
  ObjTrajNumber : Outport  Port=9
  TrajCurrentIndex : Outport  Port=10
  TrajHistBufferBValid : Outport  Port=11
  TrajHistBufferDxv : Outport  Port=12
  TrajHistBufferDyv : Outport  Port=13
  TrajHistBufferTTimeStamp : Outport  Port=14
  TrajHistBufferClass : Outport  Port=15
  EgoMove : Outport  Port=16
  wires:
  Constant7/1 -> CalcEgoVehMove/1(tCycle)
  [Get_VxvRef_ms] -> CalcEgoVehMove/3(Vego)
  [Get_AlpSideSlipAngle] -> CalcEgoVehMove/4(alpSideSlipAngle)
  [Get_KapTraj] -> CalcEgoVehMove/2(Kap)
  Constant5/1 -> CalcCompensateEgoVehMove/3(tCycle)
  Memory24/1 -> CalcCompensateEgoVehMove/8(TrajHistBufferBValidK1)
  Memory25/1 -> CalcCompensateEgoVehMove/9(TrajHistBufferDxvK1)
  Memory26/1 -> CalcCompensateEgoVehMove/10(TrajHistBufferDyvK1)
  Memory27/1 -> CalcCompensateEgoVehMove/11(TrajHistBufferTTimeStampK1)
  [EgoMove] -> Bus Selector/1
  Bus Selector/1 -> CalcCompensateEgoVehMove/4(dDeltaX)  "<dDeltaX>"
  Bus Selector/2 -> CalcCompensateEgoVehMove/5(dDeltaY)  "<dDeltaY>"
  Bus Selector/3 -> CalcCompensateEgoVehMove/6(CosOfPsi)  "<CosOfPsi>"
  Bus Selector/4 -> CalcCompensateEgoVehMove/7(SinOfPsi)  "<SinOfPsi>"
  [EgoMove] -> Bus Selector3/1
  [Get_ObjDx] -> Priority/4(ObjDx)
  [Get_ObjClass] -> Priority/3(ObjClass)
  [Get_ObjValid] -> Priority/2(ObjValid)
  ReleaseLowPriorityObjects/2(TrajHistBufferBTrajEnd) -> AssignHighPriorityObjects/13(TrajHistBufferBTrajEndK1)
  ReleaseLowPriorityObjects/1(TrajUsed) -> AssignHighPriorityObjects/12(TrajUsedK1)
  AssignHighPriorityObjects/3(ObjTrajNumber) -> ObjTrajNumber/1, [ObjTrajNumber]
  ReleaseLowPriorityObjects/3(ObjTrajNumber) -> AssignHighPriorityObjects/14(ObjTrajNumberK1)
  AssignHighPriorityObjects/1(TrajUsed) -> TrajUsed/1, [TrajUsed]
  AssignHighPriorityObjects/2(TrajHistBufferBTrajEnd) -> TrajHistBufferBTrajEnd/1, [TrajHistBufferBTrajEnd]
  AssignHighPriorityObjects/9(TrajHistBufferClass) -> Memory42/1, TrajHistBufferClass/1
  [ObjPrio] -> AssignHighPriorityObjects/5(ObjPrio)
  CalcCompensateEgoVehMove/1(TrajHistBufferBValid) -> [t_TrajHistBufferBValid]
  [t_TrajHistBufferBValid] -> AssignHighPriorityObjects/16(TrajHistBufferBValidK1)
  CalcCompensateEgoVehMove/2(TrajHistBufferDxv) -> [t_TrajHistBufferDxv]
  [t_TrajHistBufferDxv] -> AssignHighPriorityObjects/17(TrajHistBufferDxvK1)
  [t_TrajHistBufferDyv] -> AssignHighPriorityObjects/18(TrajHistBufferDyvK1)
  CalcCompensateEgoVehMove/4(TrajHistBufferTTimeStamp) -> [t_TrajHistBufferTTimeStamp]
  [t_TrajHistBufferTTimeStamp] -> AssignHighPriorityObjects/19(TrajHistBufferTTimeStampK1)
  Memory36/1 -> ReleaseLowPriorityObjects/6(TrajCurrentIndex)
  Memory37/1 -> AssignHighPriorityObjects/15(TrajCurrentIndexK1)
  Memory38/1 -> ReleaseLowPriorityObjects/8(TrajHistBufferBTrajEndK1)
  Memory40/1 -> ReleaseLowPriorityObjects/9(ObjTrajNumberK1)
  Memory41/1 -> ReleaseLowPriorityObjects/7(TrajUsedK1)
  Memory42/1 -> AssignHighPriorityObjects/20(TrajHistBufferClassK1)
  [TrajUsed] -> Memory41/1
  [ObjTrajNumber] -> Memory40/1
  [TrajHistBufferBTrajEnd] -> Memory38/1
  [ObjPrio] -> ReleaseLowPriorityObjects/3(ObjPrio)
  [Get_ObjValid] -> ReleaseLowPriorityObjects/5(ObjValid)
  AssignHighPriorityObjects/5(TrajHistBufferBValid) -> TrajHistBufferBValid/1, [TrajHistBufferBValid]
  AssignHighPriorityObjects/7(TrajHistBufferDyv) -> TrajHistBufferDyv/1, [TrajHistBufferDyv]
  AssignHighPriorityObjects/6(TrajHistBufferDxv) -> TrajHistBufferDxv/1, [TrajHistBufferDxv]
  [TrajCurrentIndex] -> Memory36/1
  [TrajCurrentIndex] -> Memory37/1
  [Get_VxvRef_ms] -> AssignHighPriorityObjects/7(VxvRef)
  [Get_ObjClass] -> AssignHighPriorityObjects/9(ObjClass)
  [Get_ObjDx] -> AssignHighPriorityObjects/10(ObjDxv)
  AssignHighPriorityObjects/4(TrajCurrentIndex) -> TrajCurrentIndex/1, [TrajCurrentIndex]
  [Get_ObjDy] -> AssignHighPriorityObjects/11(ObjDyv)
  [TrajHistBufferTTimeStamp] -> Memory27/1
  [TrajHistBufferDxv] -> Memory25/1
  [TrajHistBufferDyv] -> Memory26/1
  [TrajHistBufferBValid] -> Memory24/1
  [Get_ObjCntAlive] -> AssignHighPriorityObjects/8(ObjCntAlive)
  KapTraj/1 -> [Get_KapTraj]
  VxvRef/1 -> [Get_VxvRef_ms]
  AlpSideSlipAngle/1 -> [Get_AlpSideSlipAngle]
  Constant3/1 -> CalcCompensateEgoVehMove/1(BufNumber)
  Constant4/1 -> CalcCompensateEgoVehMove/2(TrajNumber)
  Constant13/1 -> Priority/1(ObjNumber)
  Constant15/1 -> ReleaseLowPriorityObjects/1(ObjNumber)
  Constant14/1 -> ReleaseLowPriorityObjects/2(TrajNumber)
  Constant18/1 -> AssignHighPriorityObjects/1(ObjNumber)
  Constant17/1 -> AssignHighPriorityObjects/2(TrajNumber)
  Constant16/1 -> AssignHighPriorityObjects/3(BufNumber)
  [ObjMatrix] -> ReleaseLowPriorityObjects/4(ObjMatrix)
  [ObjMatrix] -> AssignHighPriorityObjects/6(ObjMatrix)
  Constant2/1 -> StoreEgoTrajectory/1(BufNumber)
  Constant6/1 -> StoreEgoTrajectory/2(tCycle)
  StoreEgoTrajectory/7(EgoTrajHistDyv) -> EgoTrajHistDyv/1, Memory29/1
  Memory28/1 -> StoreEgoTrajectory/10(EgoTrajHistTTimeStampK1)
  Memory29/1 -> StoreEgoTrajectory/9(EgoTrajHistDyvK1)
  StoreEgoTrajectory/6(EgoTrajHistDxv) -> EgoTrajHistDxv/1, Memory30/1
  Memory30/1 -> StoreEgoTrajectory/8(EgoTrajHistDxvK1)
  StoreEgoTrajectory/5(EgoTrajHistCurrentIndex) -> EgoTrajHistCurrentIndex/1, Memory31/1
  Memory31/1 -> StoreEgoTrajectory/7(EgoTrajHistCurrentIndexK1)
  StoreEgoTrajectory/8(EgoTrajHistTTimeStamp) -> EgoTrajHistTTimeStamp/1, Memory28/1
  Bus Selector3/3 -> StoreEgoTrajectory/5(EgoCosOfPsi)  "<CosOfPsi>"
  Bus Selector3/2 -> StoreEgoTrajectory/4(EgoDDeltaY)  "<dDeltaY>"
  Bus Selector3/4 -> StoreEgoTrajectory/6(EgoSinOfPsi)  "<SinOfPsi>"
  Bus Selector3/1 -> StoreEgoTrajectory/3(EgoDDeltaX)  "<dDeltaX>"
  AssignHighPriorityObjects/8(TrajHistBufferTTimeStamp) -> TrajHistBufferTTimeStamp/1, [TrajHistBufferTTimeStamp]
  ObjValid/1 -> [Get_ObjValid]
  ObjectDy/1 -> [Get_ObjDy]
  ObjectDx/1 -> [Get_ObjDx]
  ObjectClass/1 -> [Get_ObjClass]
  ObjectCntAlive/1 -> [Get_ObjCntAlive]
  CalcEgoVehMove/1(dDeltaX) -> Bus Creator3/1  "dDeltaX"
  CalcEgoVehMove/2(dDeltaY) -> Bus Creator3/2  "dDeltaY"
  CalcEgoVehMove/3(CosOfPsi) -> Bus Creator3/3  "CosOfPsi"
  CalcEgoVehMove/4(SinOfPsi) -> Bus Creator3/4  "SinOfPsi"
  Priority/1(ObjPrio) -> ObjPrio/1, [ObjPrio]
  Priority/2(ObjMatrix) -> [ObjMatrix], ObjMatrix/1
  CalcCompensateEgoVehMove/3(TrajHistBufferDyv) -> [t_TrajHistBufferDyv]
  Constant1/1 -> CalcEgoVehMove/5(WheelTrack)
  Constant8/1 -> CalcEgoVehMove/6(Vch)
  CalcEgoVehMove/5(SlipDislim) -> [SlipDislim]
  [SlipDislim] -> AssignHighPriorityObjects/4(SlipDisLim)
  Bus Creator3/1 -> EgoMove/1, [EgoMove]
  StoreEgoTrajectory/4(Pd) -> Bus Creator3/8
  StoreEgoTrajectory/3(Pc) -> Bus Creator3/7
  StoreEgoTrajectory/2(Pb) -> Bus Creator3/6
  StoreEgoTrajectory/1(Pa) -> Bus Creator3/5

== system Noa_Nofusion/TOS2/Subsystem1/ACCOSM/ObjMatrixTransit/Subsystem/For Each Subsystem ==
  <EQ4_OBJ_ELEM> : Inport  Partition=on  PartitionDimension=1  PartitionWidth=1  PartitionOffset=0
  Bus Selector : BusSelector  OutputSignals=OBJ_ID,OBJ_Existence_Probability,OBJ_Object_Class,OBJ_Width,OBJ_Long_Distance,OBJ_Lat_Distance,OBJ_Abs_Long_Acc,OBJ_Abs_Long_Velocity,OBJ_Abs_Lat_Velocity,OBJ_Brake_Light,OBJ_Object_Age,OBJ_Motion_Status,OBJ_Motion_Category,OBJ_Motion_Orientation
  For Each : ForEach  DisableCoverage=on
  id : Outport  ConcatenationDimension=1
  confidence : Outport  Port=2  ConcatenationDimension=1
  classification : Outport  Port=3  ConcatenationDimension=1
  width : Outport  Port=4  ConcatenationDimension=1
  LongDis : Outport  Port=5  ConcatenationDimension=1
  LatDis : Outport  Port=6  ConcatenationDimension=1
  AbsLongAcc : Outport  Port=7  ConcatenationDimension=1
  AbsLongVel : Outport  Port=8  ConcatenationDimension=1
  AbsLatVel : Outport  Port=9  ConcatenationDimension=1
  BrakeLight : Outport  Port=10  ConcatenationDimension=1
  Age : Outport  Port=11  ConcatenationDimension=1
  motionSts : Outport  Port=12  ConcatenationDimension=1
  motionCategory : Outport  Port=13  ConcatenationDimension=1
  motionOrientation : Outport  Port=14  ConcatenationDimension=1
  wires:
  <EQ4_OBJ_ELEM>/1 -> Bus Selector/1
  Bus Selector/12 -> motionSts/1  "<OBJ_Motion_Status>"
  Bus Selector/6 -> LatDis/1  "<OBJ_Lat_Distance>"
  Bus Selector/9 -> AbsLatVel/1  "<OBJ_Abs_Lat_Velocity>"
  Bus Selector/7 -> AbsLongAcc/1  "<OBJ_Abs_Long_Acc>"
  Bus Selector/1 -> id/1  "<OBJ_ID>"
  Bus Selector/2 -> confidence/1  "<OBJ_Existence_Probability>"
  Bus Selector/10 -> BrakeLight/1  "<OBJ_Brake_Light>"
  Bus Selector/8 -> AbsLongVel/1  "<OBJ_Abs_Long_Velocity>"
  Bus Selector/5 -> LongDis/1  "<OBJ_Long_Distance>"
  Bus Selector/11 -> Age/1  "<OBJ_Object_Age>"
  Bus Selector/4 -> width/1  "<OBJ_Width>"
  Bus Selector/14 -> motionOrientation/1  "<OBJ_Motion_Orientation>"
  Bus Selector/3 -> classification/1  "<OBJ_Object_Class>"
  Bus Selector/13 -> motionCategory/1  "<OBJ_Motion_Category>"

== system Noa_Nofusion/TOS2/Subsystem1/ACCOSM/ObjMatrixTransit/Subsystem/For Iterator Subsystem ==
  <EQ4_OBJ_ELEM> : Inport
  Bus Selector : BusSelector  OutputSignals=OBJ_ID,OBJ_Existence_Probability,OBJ_Object_Class,OBJ_Width,OBJ_Long_Distance,OBJ_Lat_Distance,OBJ_Abs_Long_Acc,OBJ_Abs_Long_Velocity,OBJ_Abs_Lat_Velocity,OBJ_Brake_Light,OBJ_Object_Age,OBJ_Motion_Status,OBJ_Motion_Category,OBJ_Motion_Orientation
  For Iterator : ForIterator  IterationLimit=20
  Selector : Selector  InputPortWidth=20  IndexOptions=Index vector (port)  Indices=[1 3]  OutputSizes=1
  id : Outport
  confidence : Outport  Port=2
  classification : Outport  Port=3
  width : Outport  Port=4
  LongDis : Outport  Port=5
  LatDis : Outport  Port=6
  AbsLongAcc : Outport  Port=7
  AbsLongVel : Outport  Port=8
  AbsLatVel : Outport  Port=9
  BrakeLight : Outport  Port=10
  Age : Outport  Port=11
  motionSts : Outport  Port=12
  motionCategory : Outport  Port=13
  motionOrientation : Outport  Port=14
  wires:
  <EQ4_OBJ_ELEM>/1 -> Selector/1
  For Iterator/1 -> Selector/2
  Selector/1 -> Bus Selector/1
  Bus Selector/1 -> id/1  "<OBJ_ID>"
  Bus Selector/2 -> confidence/1  "<OBJ_Existence_Probability>"
  Bus Selector/3 -> classification/1  "<OBJ_Object_Class>"
  Bus Selector/4 -> width/1  "<OBJ_Width>"
  Bus Selector/5 -> LongDis/1  "<OBJ_Long_Distance>"
  Bus Selector/6 -> LatDis/1  "<OBJ_Lat_Distance>"
  Bus Selector/7 -> AbsLongAcc/1  "<OBJ_Abs_Long_Acc>"
  Bus Selector/8 -> AbsLongVel/1  "<OBJ_Abs_Long_Velocity>"
  Bus Selector/9 -> AbsLatVel/1  "<OBJ_Abs_Lat_Velocity>"
  Bus Selector/10 -> BrakeLight/1  "<OBJ_Brake_Light>"
  Bus Selector/11 -> Age/1  "<OBJ_Object_Age>"
  Bus Selector/12 -> motionSts/1  "<OBJ_Motion_Status>"
  Bus Selector/13 -> motionCategory/1  "<OBJ_Motion_Category>"
  Bus Selector/14 -> motionOrientation/1  "<OBJ_Motion_Orientation>"
